simulink model "wahdlo_model3_2015"  (R2015a)
settings: Solver=ode4  StartTime=0.0  StopTime=15  FixedStep=0.001  RelTol=1e-3
values from neighbouring files (symbols this model uses):
  A = [0 1 0 0 ... (first row only)    [Epsilon.m]
  B = [0; -m_wah*L*c2/Jr; 0; c2]    [Epsilon.m]
  C = eye(4)    [Epsilon.m]
  c1 = 5.8    [Epsilon.m]
  c2 = -18    [Epsilon.m]
  D = zeros(4,1)    [Epsilon.m]
  g = 9.81    [Epsilon.m]
  Jr = J_sm + m_wah*L^2    [Epsilon.m]
  x0 = zeros(4,1)    [Epsilon.m]
undefined symbols (not defined in the file or in its folder): K, L, m_wah, sigbuilder_block
settings Model: CovModelRefEnable=off  Creator=Mike  LastModifiedBy=Student
settings DataIOCC: LimitDataPoints=off  SaveFormat=Dataset
settings HardwareCC: ProdBitPerPointer=64  ProdLargestAtomicFloat=Float  ProdIntDivRoundTo=Zero  ProdEndianess=LittleEndian  ProdHWDeviceType=Specified
settings ModelReferenceCC: PropagateSignalLabelsOutOfModel=on

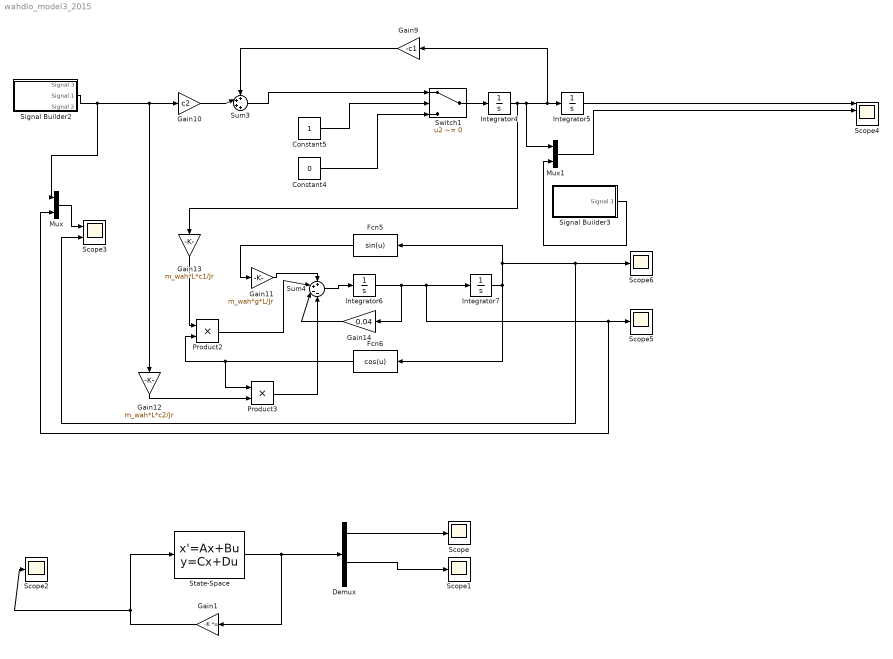
== system wahdlo_model3_2015 ==
  Constant4 : Constant  Value=0
  Constant5 : Constant
  Demux : Demux
  Fcn5 : Fcn  Expr=sin(u)
  Fcn6 : Fcn  Expr=cos(u)
  Gain1 : Gain  Gain=-K  Multiplication=Matrix(K*u) (u vector)
  Gain10 : Gain  Gain=c2
  Gain11 : Gain  Gain=m_wah*g*L/Jr
  Gain12 : Gain  Gain=m_wah*L*c2/Jr
  Gain13 : Gain  Gain=m_wah*L*c1/Jr
  Gain14 : Gain  Gain=0.04
  Gain9 : Gain  Gain=-c1
  Integrator4 : Integrator
  Integrator5 : Integrator
  Integrator6 : Integrator
  Integrator7 : Integrator  InitialCondition=pi
  Mux : Mux  Inputs=2
  Mux1 : Mux  Inputs=2
  Product2 : Product
  Product3 : Product
  Scope{,1..2,5..6} (5 alike) : Scope
      Scope settings: YMin=-0.06574  YMax=0.20123
      Scope1 settings: YMin=-0.03526  YMax=0.31735  SaveName=ScopeData2
      Scope2 settings: YMin=-0.52599  YMax=0.06854
      Scope5 settings: YMin=-6.75823  YMax=6.60568  SaveName=fi_pr_Sim
      Scope6 settings: YMin=2.14159  YMax=4.14159  SaveName=fiSim
  Scope3 : Scope  NumInputPorts=2
      settings: TickLabels=on  YMin=-5~-5  YMax=5~5  SampleInput=on
  Scope4 : Scope  NumInputPorts=4
      settings: YMin=-1.25614~-5~-5~-5  YMax=2.46205~5~5~5  SaveName=ScopeData2
  Signal Builder2 : Subsystem  Tag=STV Subsys  LoadFcn=sigbuilder_block('load',[7.5 67.5 1428 711.75 ]);  StartFcn=sigbuilder_block('start');  StopFcn=sigbuilder_block('stop');  ClipboardFcn=sigbuilder_block('clipboard');  mask(Sigbuilder block){}
      mask help: Simulink:masks:SigbuilderBlock_MD
      mask init:
      | if ~strcmp(get_param(bdroot(gcbh),'SimulationStatus'),'stopped') tuvar = sigbuilder_block('maskInit'); end
      settings: CopyFcn=sigbuilder_block('copy');  DeleteFcn=sigbuilder_block('delete');  ModelCloseFcn=sigbuilder_block('modelClose');  PreSaveFcn=sigbuilder_block('preSave');  PauseFcn=sigbuilder_block('pause');  ContinueFcn=sigbuilder_block('continue');  NameChangeFcn=sigbuilder_block('namechange');  OpenFcn=sigbuilder_block('open',[6 0 1428 711.75 ]);  CloseFcn=sigbuilder_block('close');
      mask Display: plot(0, 0, 100, 100,[2, 2, 32, 32, 2], [68, 8, 8, 68, 68],[32, 2], [38, 38], [32, 19, 2],[53, 60, 44], [32, 17, 17, 2],[16, 16, 31, 31]);txt = getActiveGroup(gcbh);text(2, 100, txt,'verticalAlignment', 'top');
  Signal Builder3 : Subsystem  Tag=STV Subsys  LoadFcn=sigbuilder_block('load');  StartFcn=sigbuilder_block('start');  StopFcn=sigbuilder_block('stop');  ClipboardFcn=sigbuilder_block('clipboard');  mask(Sigbuilder block){}
      mask help: Simulink:masks:SigbuilderBlock_MD
      mask init:
      | if ~strcmp(get_param(bdroot(gcbh),'SimulationStatus'),'stopped') tuvar = sigbuilder_block('maskInit'); end
      settings: CopyFcn=sigbuilder_block('copy');  DeleteFcn=sigbuilder_block('delete');  ModelCloseFcn=sigbuilder_block('modelClose');  PreSaveFcn=sigbuilder_block('preSave');  PauseFcn=sigbuilder_block('pause');  ContinueFcn=sigbuilder_block('continue');  NameChangeFcn=sigbuilder_block('namechange');  OpenFcn=sigbuilder_block('open',[437.6 199.2 550.4 400 ]);  CloseFcn=sigbuilder_block('close');
      mask Display: plot(0, 0, 100, 100,[2, 2, 32, 32, 2], [68, 8, 8, 68, 68],[32, 2], [38, 38], [32, 19, 2],[53, 60, 44], [32, 17, 17, 2],[16, 16, 31, 31]);txt = getActiveGroup(gcbh);text(2, 100, txt,'verticalAlignment', 'top');
  State-Space : StateSpace  A=A  B=B  C=C  D=D  X0=x0+[pi/18;0;0;0]
  Sum3 : Sum  Inputs=4
  Sum4 : Sum  Inputs=++--
  Switch1 : Switch  Criteria=u2 ~= 0
  wires:
  Integrator4/1 -> Gain13/1, Mux1/1, Gain9/1, Integrator5/1
  Sum3/1 -> Switch1/1
  Gain9/1 -> Sum3/1
  Gain10/1 -> Sum3/2
  Signal Builder3/1(Signal 3) -> Mux1/2
  Integrator5/1 -> Scope4/1
  Mux1/1 -> Scope4/2
  Integrator6/1 -> Gain14/1, Mux/2, Scope5/1, Integrator7/1
  Gain11/1 -> Sum4/1
  Integrator7/1 -> Fcn6/1, Scope3/2, Scope6/1, Fcn5/1
  Fcn5/1 -> Gain11/1
  Fcn6/1 -> Product3/1, Product2/2
  Product2/1 -> Sum4/2
  Gain13/1 -> Product2/1
  Signal Builder2/2(Signal 1) -> Mux/1, Gain12/1, Gain10/1
  Gain14/1 -> Sum4/3
  Sum4/1 -> Integrator6/1
  Switch1/1 -> Integrator4/1
  Constant4/1 -> Switch1/3
  Constant5/1 -> Switch1/2
  Gain12/1 -> Product3/2
  Product3/1 -> Sum4/4
  State-Space/1 -> Gain1/1, Demux/1
  Demux/1 -> Scope/1
  Demux/3 -> Scope1/1
  Gain1/1 -> Scope2/1, State-Space/1
  Mux/1 -> Scope3/1

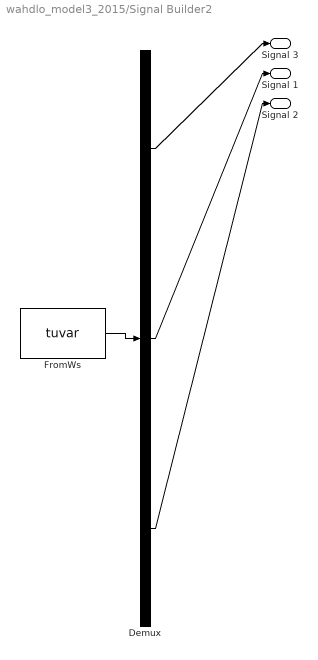
== system wahdlo_model3_2015/Signal Builder2 ==
  Demux : Demux  Tag=STV Demux  Outputs=3
  FromWs : FromWorkspace  Tag=STV FromWs  VariableName=tuvar  SampleTime=0
      SigBuilderData=|
      | common.afterFinalStr = 'Extrapolate'
      | common.sampleTime = 0
      | dataSet.timeRange = [0 30]
      | dataSet.name = 'Group 1'
      | sbobj.Groups.Name = 'Group 1'
      | sbobj.Groups.Signals(1).Name = 'Signal 3'
      | sbobj.Groups.Signals(1).XData = [0 0.01 0.02 0.03 0.04 0.05 0.06 0.07 0.08 0.09 0.1 0.11 ... (3001 elements, 1x3001)]
      | sbobj.Groups.Signals(1).YData = [0.1 0.1 0.1 0.1 0.1 0.1 0.1 0.1 0.1 0.1 0.1 0.1 ... (3001 elements, 1x3001)]
      | sbobj.Groups.Signals(2).Name = 'Signal 1'
      | sbobj.Groups.Signals(2).XData = [0 0.01 0.02 0.03 0.04 0.05 0.06 0.07 0.08 0.09 0.1 0.11 ... (3001 elements, 1x3001)]
      | sbobj.Groups.Signals(2).YData = [0 0 0 0 0 0 0 0 0 0 0 0 ... (3001 elements, 1x3001)]
      | sbobj.Groups.Signals(3).Name = 'Signal 2'
      | sbobj.Groups.Signals(3).XData = [0 0.43 0.43 1 1 1.78 1.78 2.54 2.54 6 7 8 8 9 10 10 11 11 12 12 13 13 14 14 15 15 16 16 17 17 18 18 19 19 20 20 21 21 22 22 23 23 24 24 25 25 26 26 27 27 28 28 29 29 30]
      | sbobj.Groups.Signals(3).YData = [0.5 0.5 -0.5 -0.5 0.46 0.46 -0.5 -0.5 0.005 0.005 0.005 0.005 0.01 0.01 0.01 0.5 0.5 -0.5 -0.5 0.5 0.5 -0.5 -0.5 0.5 0.5 -0.5 -0.5 0.5 0.5 -0.5 -0.5 0.5 0.5 -0.5 -0.5 0.5 0.5 -0.5 -0.5 0.5 0.5 -0.5 -0.5 0.5 0.5 -0.5 -0.5 0.5 0.5 -0.5 -0.5 0.5 0.5 -0.5 -0.5]
      | sbobj.Groups.TimeRange = [0 30]
  Signal 3 : Outport  Tag=STV Outport
  Signal 1 : Outport  Tag=STV Outport  Port=2
  Signal 2 : Outport  Tag=STV Outport  Port=3
  wires:
  FromWs/1 -> Demux/1
  Demux/1 -> Signal 3/1
  Demux/2 -> Signal 1/1
  Demux/3 -> Signal 2/1

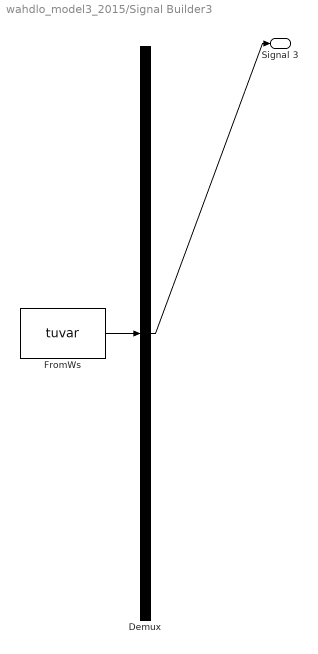
== system wahdlo_model3_2015/Signal Builder3 ==
  Demux : Demux  Tag=STV Demux  Outputs=1
  FromWs : FromWorkspace  Tag=STV FromWs  VariableName=tuvar  SampleTime=0
      SigBuilderData=|
      | common.afterFinalStr = 'Extrapolate'
      | common.sampleTime = 0
      | dataSet.timeRange = [0 30]
      | dataSet.name = 'Group 1'
      | sbobj.Groups.Name = 'Group 1'
      | sbobj.Groups.Signals.Name = 'Signal 3'
      | sbobj.Groups.Signals.XData = [0 0.01 0.02 0.03 0.04 0.05 0.06 0.07 0.08 0.09 0.1 0.11 ... (3001 elements, 1x3001)]
      | sbobj.Groups.Signals.YData = [2.0902351 0 -0.0057053 -0.0114106 -0.0171159 -0.0171159 -0.0171159 -0.0171159 -0.0171159 -0.0114106 -0.0114106 -0.0114106 ... (3001 elements, 1x3001)]
      | sbobj.Groups.TimeRange = [0 30]
  Signal 3 : Outport  Tag=STV Outport
  wires:
  FromWs/1 -> Demux/1
  Demux/1 -> Signal 3/1
